simulink model "lss"  (R2022b)
settings: Solver=FixedStepAuto  StartTime=0.0  StopTime=Inf  FixedStep=0.001  RelTol=1e-3  EnableMultiTasking=on
InitFcn:
  | clear mex
model workspace (MAT data in the model file):
  worldsim_instance.endpoint_ip = '127.0.0.1'
  worldsim_instance.endpoint_port = 8080
values from neighbouring files (symbols this model uses):
  ADAS_Control_Mode = 1    [LSS_parameters.m]    (also in lss_ini_param.sldd = 1.0)
  butter_a = 1.0 -1.9911142922016536 0.99115359586893548    [lss_ini_param.sldd]
  butter_a_lka_out = 1.0 -1.5610180758007179 0.641351538057563    [lss_ini_param.sldd]
  butter_b = 9.825916820482009E-6 1.9651833640964018E-5 9.825916820482009E-6    [lss_ini_param.sldd]
  butter_b_lka_out = 0.020083365564211246 0.040166731128422492 0.020083365564211246    [lss_ini_param.sldd]
  index_variant_approaching_speed = 3.0    [lss_ini_param.sldd]
  initCond = vi_worldsim_load_scenario(worldsim_process,scenario_path,'lss_online')    [launcher.m]
  LDW_Activity_Flag = 1    [LSS_parameters.m]    (also in lss_ini_param.sldd = 1.0)
  LDW_Freq_Hz = Sensor_Freq_worldsim    [LSS_parameters.m]    (also in lss_ini_param.sldd = 50.0)
  LDW_LaneGap_dydt_Warning = 50    [LSS_parameters.m]    (also in lss_ini_param.sldd = 50.0)
  LDW_LaneGap_Warning = [0.5 0.25]    [LSS_parameters.m]    (also in lss_ini_param.sldd = 0.5 0.25)
  LDW_Min_Speed = 60    [LSS_parameters.m]    (also in lss_ini_param.sldd = 60.0)
  LDW_Steer_Vibration_Amplitude = 5    [LSS_parameters.m]    (also in lss_ini_param.sldd = 5.0)
  LDW_Steer_Vibration_Freq = 25    [LSS_parameters.m]    (also in lss_ini_param.sldd = 25.0)
  LKA_Activity_Flag = 1    [LSS_parameters.m]    (also in lss_ini_param.sldd = 1.0)
  LKA_D = [0.2 0.3]    [LSS_parameters.m]    (also in lss_ini_param.sldd = 0.2 0.3)
  LKA_Dyn_Rate_Limiter_Gain = 0.1    [LSS_parameters.m]    (also in lss_ini_param.sldd)
  LKA_Dyn_Rate_Limiter_Power = 10    [LSS_parameters.m]    (also in lss_ini_param.sldd = 10.0)
  LKA_Error_dydt_Off = 1    [LSS_parameters.m]    (also in lss_ini_param.sldd = 1.0)
  LKA_Error_Max = 3    [LSS_parameters.m]    (also in lss_ini_param.sldd = 3.0)
  LKA_Error_Off = 0.5    [LSS_parameters.m]    (also in lss_ini_param.sldd)
  LKA_Freq_Hz = Sensor_Freq_worldsim    [LSS_parameters.m]    (also in lss_ini_param.sldd = 50.0)
  LKA_I = [0.025 0.05]    [LSS_parameters.m]    (also in lss_ini_param.sldd = 0.025 0.05)
  LKA_Lane_Gap_Activate = [0.25 0.125]    [LSS_parameters.m]    (also in lss_ini_param.sldd = -0.05 0.125)
  LKA_Lane_Gap_dydt_Activate = 50    [LSS_parameters.m]    (also in lss_ini_param.sldd = 50.0)
  LKA_Min_Speed = 60    [LSS_parameters.m]    (also in lss_ini_param.mat = 50; lss_ini_param.sldd = 50.0)
  LKA_On_Display_Freq = 5    [LSS_parameters.m]    (also in lss_ini_param.sldd = 5.0)
  LKA_P = [0.1 0.2]    [LSS_parameters.m]    (also in lss_ini_param.sldd = 0.1 0.2)
  LKA_Steer_Rate_Max_radps = 1    [LSS_parameters.m]    (also in lss_ini_param.sldd = 1.0)
  radar_source = 2    [LSS_parameters.m]    (also in lss_ini_param.sldd = 2.0)
  Sensor_Freq_worldsim = 50    [launcher.m]    (also in lss_ini_param.sldd = 50.0)
  simulation_crt = '../VI-CarRealTime_model/SedanCar_WorldSim_Offline_send_svm.xml'    [launcher.m]
  stop_number_collisions = 5    [launcher.m]
  stop_speed = 0.001    [launcher.m]
  stop_time = 20    [launcher.m]
  target_speed = 72    [LSS_parameters.m]    (also in launcher.m = initCond.initialVelocity * 3.6)
  variant_approaching_speed = v_lat    [launcher.m]    (also in lss_ini_param.sldd = 0.2 0.3 0.4 0.5 0.6)
  vehicle_width = 1.86    [LSS_parameters.m]    (also in lss_ini_param.sldd = 2.05)
undefined symbols (not defined in the file or in its folder): Driver_Demands, light_brake_center, light_brake_left, light_brake_right, steer_assist, vicrt_initcallback, vicrt_initmexcallback, vicrt_simulationmanager
libraries: simulink x39, simwbSfunlib x15, viworldsim_lib x5
(part 1 of 6)
settings Model: Creator=mcava  LastModifiedBy=pumpaipa
settings SolverCC: AlgebraicLoopSolver=TrustRegion  AutoInsertRateTranBlk=on
settings DataIOCC: LimitDataPoints=on  SaveFormat=Array  ReturnWorkspaceOutputs=off  SignalLoggingName=sigsOut
settings OptimizationCC: ExpressionDepthLimit=2147483647  InitFltsAndDblsToZero=on  LifeSpan=inf
settings DebuggingCC: SignalInfNanChecking=warning  UnderspecifiedInitializationDetection=Classic  MergeDetectMultiDrivingBlocksExec=none  SignalResolutionControl=TryResolveAllWithWarning  MultiTaskDSMMsg=warning  MultiTaskCondExecSysMsg=none  FcnCallInpInsideContextMsg=warning  UnconnectedInputMsg=warning  UnconnectedOutputMsg=warning  UnconnectedLineMsg=warning  StateNameClashWarn=warning  SFUnexpectedBacktrackingDiag=warning  SFNoUnconditionalDefaultTransitionDiag=warning  SFExecutionAtInitializationDiag=none  SFMachineParentedDataDiag=warning  ArithmeticOperatorsInVariantConditions=warning
settings HardwareCC: ProdBitPerPointer=32  ProdBitPerSizeT=32  ProdBitPerPtrDiffT=32  ProdLargestAtomicFloat=None  ProdIntDivRoundTo=Undefined  ProdEndianess=Unspecified  ProdWordSize=32  ProdHWDeviceType=32-bit Generic  TargetHWDeviceType=32-bit Generic  TargetUnknown=on  ProdEqTarget=off
settings ModelReferenceCC: EnableRefExpFcnMdlSchedulingChecks=on  PropagateSignalLabelsOutOfModel=off
settings SFSimCC: SimUseLocalCustomCode=off  CustomCodeUndefinedFunction=UseInterfaceOnly
settings RTWCC: RTWUseLocalCustomCode=off
settings CodeAppCC: StateflowObjectComments=on
settings GRTTargetCC: TargetFcnLib=ansi_tfl_tmw.mat  TargetLangStandard=C89/C90 (ANSI)  CombineOutputUpdateFcns=off  GRTInterface=on
settings ConfigComp: CovMetricSettings=dw  CovSaveCumulativeToWorkspaceVar=on  CovSaveSingleToWorkspaceVar=on  CovExternalEMLEnable=off

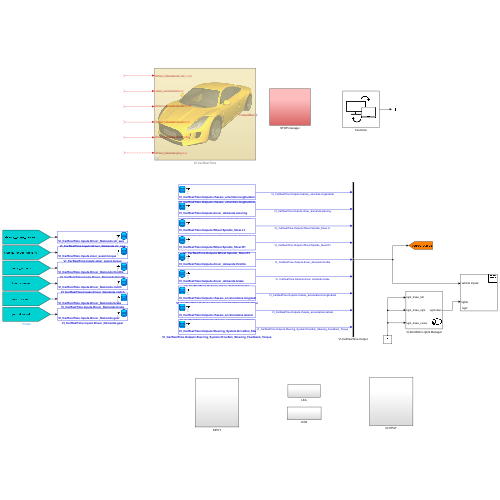
[thumbnail: Simulink's stored preview of the top-level diagram]
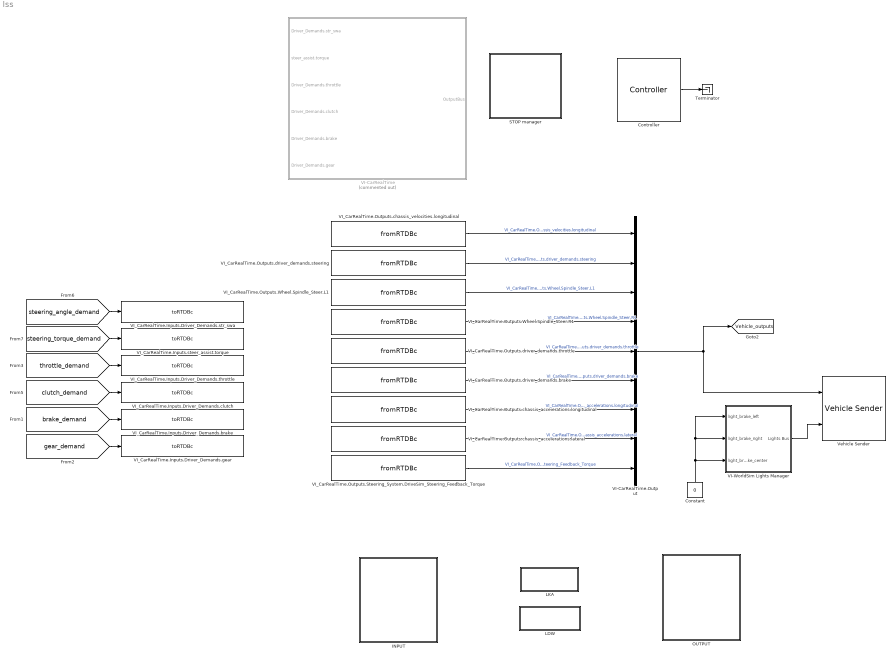
== system lss ==
  Constant : Constant  Value=0
  Controller : viworldsim_lib/Controller  worldsim_endpoint_ip=worldsim_instance.endpoint_ip  worldsim_endpoint_port=worldsim_instance.endpoint_port  worldsim_verbose=off
  INPUT : Subsystem
  LDW : Subsystem
  LKA : Subsystem
  OUTPUT : Subsystem
  STOP manager : Subsystem
  Terminator : Terminator
  VI-CarRealTime : Subsystem  Commented=on  InitFcn=vicrt_simulationmanager(0);  TreatAsAtomicUnit=on  mask{useOutputMapInMaskFlag=on}
      mask prompts: useOutputMapInMaskFlag "Output Port Names From Output Map"
      mask help: Full VI-CarRealTime mex integrated with IO Bus
      settings: CopyFcn=set_param(gcb, 'LinkStatus', 'none');  ModelCloseFcn=vicrt_simulationmanager(2);  OpenFcn=vicrt_simulationmanager(1);
      mask Display: image(imread('vehicle.jpg'));color('red');port_label('input',1,'Driver_Demands.str_swa');port_label('input',2,'steer_assist.torque');port_label('input',3,'Driver_Demands.throttle');port_label('input',4,'Driver_Demands.clutch');port_label('input',5,'Driver_Demands.brake');port_label('input',6,'Driver_Demands.gear');port_label('output',1,'OutputBus');
  VI-CarRealTime.Output : BusCreator  Inputs=9
  VI-WorldSim Lights Manager : Subsystem  mask{DummyMaskPar=0}
      mask init:
      | set_param(gcb, 'LinkStatus','none')
      settings: OpenFcn=|
      | wsoffline_lightsmanager;
      | set_param(gcb, 'LinkStatus','none');
      mask Display:
      | color('black');
      | image('lights.png', [85 0 50 50]);
  VI_CarRealTime.Inputs.Driver_Demands.brake : simwbSfunlib/toRTDBc  stringBlock=off  varName=VI_CarRealTime.Inputs.Driver_Demands.brake  sigDim=[1 1]  sigType=double  sampleTime=[-1 0]  maxBuffSize=1024  busName=nobus  defaultValue=0  defaultString=simwbout  hasMapping=0  ptrName=VI_CarRealTime_Inputs_Driver_Demands_brake  enumOrAlias=nothing
      settings: SourceProductName=SimWB MLToolkit
  VI_CarRealTime.Inputs.Driver_Demands.clutch : simwbSfunlib/toRTDBc  stringBlock=off  varName=VI_CarRealTime.Inputs.Driver_Demands.clutch  sigDim=[1 1]  sigType=double  sampleTime=[-1 0]  maxBuffSize=1024  busName=nobus  defaultValue=0  defaultString=simwbout  hasMapping=0  ptrName=VI_CarRealTime_Inputs_Driver_Demands_clutch  enumOrAlias=nothing
      settings: SourceProductName=SimWB MLToolkit
  VI_CarRealTime.Inputs.Driver_Demands.gear : simwbSfunlib/toRTDBc  stringBlock=off  varName=VI_CarRealTime.Inputs.Driver_Demands.gear  sigDim=[1 1]  sigType=double  sampleTime=[-1 0]  maxBuffSize=1024  busName=nobus  defaultValue=0  defaultString=simwbout  hasMapping=0  ptrName=VI_CarRealTime_Inputs_Driver_Demands_gear  enumOrAlias=nothing
      settings: SourceProductName=SimWB MLToolkit
  VI_CarRealTime.Inputs.Driver_Demands.str_swa : simwbSfunlib/toRTDBc  stringBlock=off  varName=VI_CarRealTime.Inputs.Driver_Demands.str_swa  sigDim=[1 1]  sigType=double  sampleTime=[-1 0]  maxBuffSize=1024  busName=nobus  defaultValue=0  defaultString=simwbout  hasMapping=0  ptrName=VI_CarRealTime_Inputs_Driver_Demands_str_swa  enumOrAlias=nothing
      settings: SourceProductName=SimWB MLToolkit
  VI_CarRealTime.Inputs.Driver_Demands.throttle : simwbSfunlib/toRTDBc  stringBlock=off  varName=VI_CarRealTime.Inputs.Driver_Demands.throttle  sigDim=[1 1]  sigType=double  sampleTime=[-1 0]  maxBuffSize=1024  busName=nobus  defaultValue=0  defaultString=simwbout  hasMapping=0  ptrName=VI_CarRealTime_Inputs_Driver_Demands_throttle  enumOrAlias=nothing
      settings: SourceProductName=SimWB MLToolkit
  VI_CarRealTime.Inputs.steer_assist.torque : simwbSfunlib/toRTDBc  stringBlock=off  varName=VI_CarRealTime.Inputs.steer_assist.torque  sigDim=[1 1]  sigType=double  sampleTime=[-1 0]  maxBuffSize=1024  busName=nobus  defaultValue=0  defaultString=simwbout  hasMapping=0  ptrName=VI_CarRealTime_Inputs_Driver_Demands_user_input_steering  enumOrAlias=nothing
      settings: SourceProductName=SimWB MLToolkit
  VI_CarRealTime.Outputs.Steering_System.DriveSim_Steering_Feedback_Torque : simwbSfunlib/fromRTDBc  stringBlock=off  varName=VI_CarRealTime.Outputs.Steering_System.DriveSim_Steering_Feedback_Torque  sigDim=[1 1]  sigType=double  sampleTime=[-1 0]  maxBuffSize=1024  busName=nobus  defaultValue=0  defaultString=simwbin  hasMapping=0  ptrName=VI_CarRealTime_Outputs_Steering_System_DriveSim_Steering_Feedback_Torque  enumOrAlias=nothing
      settings: SourceProductName=SimWB MLToolkit
  VI_CarRealTime.Outputs.Wheel.Spindle_Steer.L1 : simwbSfunlib/fromRTDBc  stringBlock=off  varName=VI_CarRealTime.Outputs.Wheel.Spindle_Steer.L1  sigDim=[1 1]  sigType=double  sampleTime=[-1 0]  maxBuffSize=1024  busName=nobus  defaultValue=0  defaultString=simwbin  hasMapping=0  ptrName=VI_CarRealTime_Outputs_Wheel_Spindle_Steer_L1  enumOrAlias=nothing
      settings: SourceProductName=SimWB MLToolkit
  VI_CarRealTime.Outputs.Wheel.Spindle_Steer.R1 : simwbSfunlib/fromRTDBc  stringBlock=off  varName=VI_CarRealTime.Outputs.Wheel.Spindle_Steer.R1  sigDim=[1 1]  sigType=double  sampleTime=[-1 0]  maxBuffSize=1024  busName=nobus  defaultValue=0  defaultString=simwbin  hasMapping=0  ptrName=VI_CarRealTime_Outputs_Wheel_Spindle_Steer_R1  enumOrAlias=nothing
      settings: SourceProductName=SimWB MLToolkit
  VI_CarRealTime.Outputs.chassis_accelerations.lateral : simwbSfunlib/fromRTDBc  stringBlock=off  varName=VI_CarRealTime.Outputs.chassis_accelerations.lateral  sigDim=[1 1]  sigType=double  sampleTime=[-1 0]  maxBuffSize=1024  busName=nobus  defaultValue=0  defaultString=simwbin  hasMapping=0  ptrName=VI_CarRealTime_Outputs_chassis_accelerations_lateral  enumOrAlias=nothing
      settings: SourceProductName=SimWB MLToolkit
  VI_CarRealTime.Outputs.chassis_accelerations.longitudinal : simwbSfunlib/fromRTDBc  stringBlock=off  varName=VI_CarRealTime.Outputs.chassis_accelerations.longitudinal  sigDim=[1 1]  sigType=double  sampleTime=[-1 0]  maxBuffSize=1024  busName=nobus  defaultValue=0  defaultString=simwbin  hasMapping=0  ptrName=VI_CarRealTime_Outputs_chassis_accelerations_longitudinal  enumOrAlias=nothing
      settings: SourceProductName=SimWB MLToolkit
  VI_CarRealTime.Outputs.chassis_velocities.longitudinal : simwbSfunlib/fromRTDBc  stringBlock=off  varName=VI_CarRealTime.Outputs.chassis_velocities.longitudinal  sigDim=[1 1]  sigType=double  sampleTime=[-1 0]  maxBuffSize=1024  busName=nobus  defaultValue=0  defaultString=simwbin  hasMapping=0  ptrName=VI_CarRealTime_Outputs_chassis_velocities_longitudinal  enumOrAlias=nothing
      settings: SourceProductName=SimWB MLToolkit
  VI_CarRealTime.Outputs.driver_demands.brake : simwbSfunlib/fromRTDBc  stringBlock=off  varName=VI_CarRealTime.Outputs.driver_demands.brake  sigDim=[1 1]  sigType=double  sampleTime=[-1 0]  maxBuffSize=1024  busName=nobus  defaultValue=0  defaultString=simwbin  hasMapping=0  ptrName=VI_CarRealTime_Outputs_driver_demands_brake  enumOrAlias=nothing
      settings: SourceProductName=SimWB MLToolkit
  VI_CarRealTime.Outputs.driver_demands.steering : simwbSfunlib/fromRTDBc  stringBlock=off  varName=VI_CarRealTime.Outputs.driver_demands.steering  sigDim=[1 1]  sigType=double  sampleTime=[-1 0]  maxBuffSize=1024  busName=nobus  defaultValue=0  defaultString=simwbin  hasMapping=0  ptrName=VI_CarRealTime_Outputs_driver_demands_steering  enumOrAlias=nothing
      settings: SourceProductName=SimWB MLToolkit
  VI_CarRealTime.Outputs.driver_demands.throttle : simwbSfunlib/fromRTDBc  stringBlock=off  varName=VI_CarRealTime.Outputs.driver_demands.throttle  sigDim=[1 1]  sigType=double  sampleTime=[-1 0]  maxBuffSize=1024  busName=nobus  defaultValue=0  defaultString=simwbin  hasMapping=0  ptrName=VI_CarRealTime_Outputs_driver_demands_throttle  enumOrAlias=nothing
      settings: SourceProductName=SimWB MLToolkit
  Vehicle Sender : viworldsim_lib/VI-WorldSim Vehicle Senders/Vehicle Sender  useOutputMapInMaskFlag=on  worldsim_car_name='ego'  worldsim_ai_controlled=off
  tag scope: Vehicle_outputs=global
  wires:
  VI-CarRealTime.Output/1 -> Vehicle Sender/1, [Vehicle_outputs]
  ? -> VI-CarRealTime/4(Driver_Demands.clutch)
  ? -> VI-CarRealTime/5(Driver_Demands.brake)
  ? -> VI-CarRealTime/2(steer_assist.torque)
  ? -> VI-CarRealTime/6(Driver_Demands.gear)
  ? -> VI-CarRealTime/3(Driver_Demands.throttle)
  ? -> VI-CarRealTime/1(Driver_Demands.str_swa)
  Controller/1 -> Terminator/1
  Constant/1 -> VI-WorldSim Lights Manager/3(light_brake_center), VI-WorldSim Lights Manager/2(light_brake_right), VI-WorldSim Lights Manager/1(light_brake_left)
  VI-WorldSim Lights Manager/1(Lights Bus) -> Vehicle Sender/2
  [steering_angle_demand] -> VI_CarRealTime.Inputs.Driver_Demands.str_swa/1
  [steering_torque_demand] -> VI_CarRealTime.Inputs.steer_assist.torque/1
  [throttle_demand] -> VI_CarRealTime.Inputs.Driver_Demands.throttle/1
  [clutch_demand] -> VI_CarRealTime.Inputs.Driver_Demands.clutch/1
  [brake_demand] -> VI_CarRealTime.Inputs.Driver_Demands.brake/1
  [gear_demand] -> VI_CarRealTime.Inputs.Driver_Demands.gear/1
  VI_CarRealTime.Outputs.Wheel.Spindle_Steer.R1/1 -> VI-CarRealTime.Output/4  "VI_CarRealTime.Outputs.Wheel.Spindle_Steer.R1"
  VI_CarRealTime.Outputs.chassis_velocities.longitudinal/1 -> VI-CarRealTime.Output/1  "VI_CarRealTime.Outputs.chassis_velocities.longitudinal"
  VI_CarRealTime.Outputs.Steering_System.DriveSim_Steering_Feedback_Torque/1 -> VI-CarRealTime.Output/9  "VI_CarRealTime.Outputs.Steering_System.DriveSim_Steering_Feedback_Torque"
  VI_CarRealTime.Outputs.chassis_accelerations.lateral/1 -> VI-CarRealTime.Output/8  "VI_CarRealTime.Outputs.chassis_accelerations.lateral"
  VI_CarRealTime.Outputs.driver_demands.brake/1 -> VI-CarRealTime.Output/6  "VI_CarRealTime.Outputs.driver_demands.brake"
  VI_CarRealTime.Outputs.Wheel.Spindle_Steer.L1/1 -> VI-CarRealTime.Output/3  "VI_CarRealTime.Outputs.Wheel.Spindle_Steer.L1"
  VI_CarRealTime.Outputs.driver_demands.throttle/1 -> VI-CarRealTime.Output/5  "VI_CarRealTime.Outputs.driver_demands.throttle"
  VI_CarRealTime.Outputs.driver_demands.steering/1 -> VI-CarRealTime.Output/2  "VI_CarRealTime.Outputs.driver_demands.steering"
  VI_CarRealTime.Outputs.chassis_accelerations.longitudinal/1 -> VI-CarRealTime.Output/7  "VI_CarRealTime.Outputs.chassis_accelerations.longitudinal"

== system lss/INPUT ==
  Inputs for CRT : Subsystem
  finalizing controls inputs : Subsystem
  simple_cruise_control : Subsystem

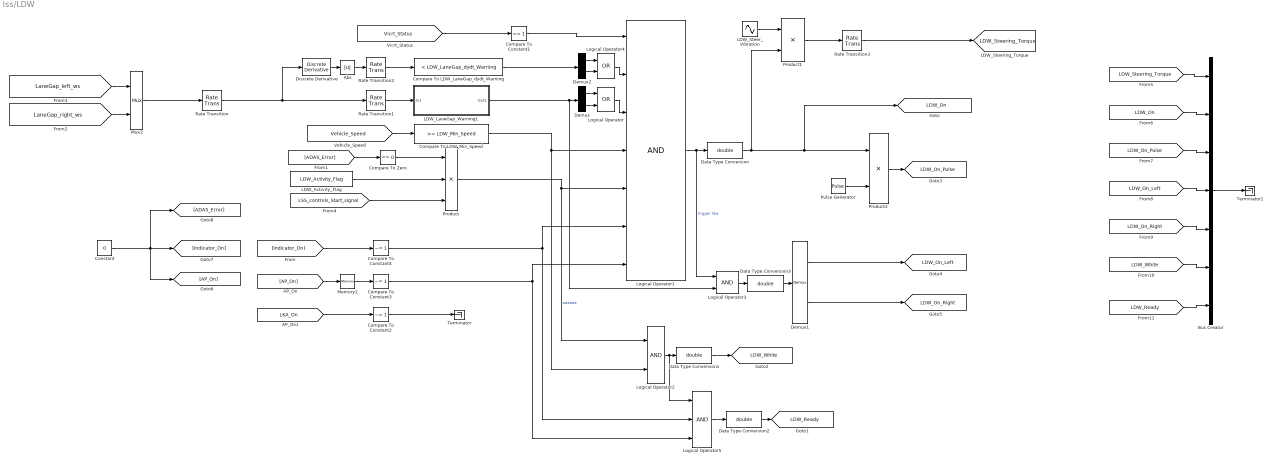
== system lss/LDW ==
  Abs : Abs  SaturateOnIntegerOverflow=off
  Bus Creator : BusCreator  Inputs=7
  Compare To Constant1 : simulink/Logic and Bit Operations/Compare To Constant  relop===  const=1  OutDataTypeStr=boolean
  Compare To Constant2 : simulink/Logic and Bit Operations/Compare To Constant  relop=~=  const=1  OutDataTypeStr=boolean
  Compare To Constant3 : simulink/Logic and Bit Operations/Compare To Constant  relop=~=  const=1  OutDataTypeStr=boolean
  Compare To Constant4 : simulink/Logic and Bit Operations/Compare To Constant  relop=~=  const=1  OutDataTypeStr=boolean
  Compare To Zero : simulink/Logic and Bit Operations/Compare To Zero  relop===  OutDataTypeStr=boolean
  Compare To LDW_LaneGap_dydt_Warning : simulink/Logic and Bit Operations/Compare To Constant  relop=<  const=LDW_LaneGap_dydt_Warning  OutDataTypeStr=boolean
  Compare To LDW_Min_Speed : simulink/Logic and Bit Operations/Compare To Constant  relop=>=  const=LDW_Min_Speed  OutDataTypeStr=boolean
  Constant : Constant  Value=0
  Data Type Conversion{,1..3} (4 alike) : DataTypeConversion  OutDataTypeStr=double  SaturateOnIntegerOverflow=off  RndMeth=Floor
  Demux : Demux  Outputs=2
  Demux1 : Demux  Outputs=2
  Demux2 : Demux  Outputs=2
  Discrete Derivative : simulink/Discrete/Discrete Derivative  gainval=1.0  ICPrevScaledInput=0.0  OutMin=[]  OutMax=[]  OutDataType=fixdt(1, 16)  OutScaling=2^-10  DoSatur=off
  LDW_Activity_Flag : Constant  Value=LDW_Activity_Flag
  LDW_LaneGap_Warning1 : Subsystem
  LDW_Steer_Vibration : Sin  Amplitude=LDW_Steer_Vibration_Amplitude  Frequency=LDW_Steer_Vibration_Freq*2*pi  SampleTime=0
  Logical Operator : Logic  Operator=OR  AllPortsSameDT=off  OutDataTypeStr=boolean
  Logical Operator1 : Logic  Inputs=7  AllPortsSameDT=off  OutDataTypeStr=boolean
  Logical Operator2 : Logic  AllPortsSameDT=off  OutDataTypeStr=boolean
  Logical Operator3 : Logic  AllPortsSameDT=off  OutDataTypeStr=boolean
  Logical Operator4 : Logic  Operator=OR  AllPortsSameDT=off  OutDataTypeStr=boolean
  Logical Operator5 : Logic  Inputs=3  AllPortsSameDT=off  OutDataTypeStr=boolean
  Memory2 : Memory
  Mux3 : Mux  Inputs=2
  Product : Product  Inputs=3
  Product1 : Product
  Product2 : Product
  Pulse Generator : DiscretePulseGenerator  PulseType=Time based  Period=1/LKA_On_Display_Freq  PulseWidth=50
  Rate Transition : RateTransition  OutPortSampleTime=1/LDW_Freq_Hz
  Rate Transition1 : RateTransition  OutPortSampleTime=1/1000
  Rate Transition2 : RateTransition  OutPortSampleTime=1/1000
  Rate Transition3 : RateTransition  OutPortSampleTime=1/1000
  Terminator : Terminator
  Terminator1 : Terminator
  tag scope: LDW_On=global, LDW_On_Left=global, LDW_On_Pulse=global, LDW_On_Right=global, LDW_Ready=global, LDW_Steering_Torque=global, LDW_White=global
  wires:
  [Vicrt_Status] -> Compare To Constant1/1
  Compare To Constant1/1 -> Logical Operator1/1
  Logical Operator1/1 -> Logical Operator3/1, Data Type Conversion/1  "trigger ldw"
  [Vehicle_Speed] -> Compare To LDW_Min_Speed/1
  Compare To LDW_Min_Speed/1 -> Logical Operator2/2, Logical Operator1/4
  Logical Operator/1 -> Logical Operator1/3
  LDW_Steer_Vibration/1 -> Product1/1
  Product1/1 -> Rate Transition3/1
  Data Type Conversion/1 -> Product2/1, [LDW_On], Product1/2
  Logical Operator2/1 -> Logical Operator5/1, Data Type Conversion1/1
  Data Type Conversion1/1 -> [LDW_White]
  Demux/1 -> Logical Operator/1
  Demux/2 -> Logical Operator/2
  Demux1/1 -> [LDW_On_Left]
  Demux1/2 -> [LDW_On_Right]
  Data Type Conversion3/1 -> Demux1/1
  Logical Operator3/1 -> Data Type Conversion3/1
  Rate Transition/1 -> Rate Transition1/1, Discrete Derivative/1
  Discrete Derivative/1 -> Abs/1
  Rate Transition2/1 -> Compare To LDW_LaneGap_dydt_Warning/1
  Compare To LDW_LaneGap_dydt_Warning/1 -> Demux2/1
  Logical Operator4/1 -> Logical Operator1/2
  Demux2/1 -> Logical Operator4/1
  Demux2/2 -> Logical Operator4/2
  Abs/1 -> Rate Transition2/1
  [Indicator_On] -> Compare To Constant4/1
  Compare To Constant4/1 -> Logical Operator1/6, Logical Operator5/2
  Logical Operator5/1 -> Data Type Conversion2/1
  Product/1 -> Logical Operator2/1, Logical Operator1/5  "aaaaaa"
  [ADAS_Error] -> Compare To Zero/1
  Compare To Zero/1 -> Product/1
  LDW_Activity_Flag/1 -> Product/2
  LDW_LaneGap_Warning1/1(Out1) -> Logical Operator3/2, Demux/1
  Rate Transition1/1 -> LDW_LaneGap_Warning1/1(In1)
  [AP_On] -> Memory2/1
  Memory2/1 -> Compare To Constant3/1
  Compare To Constant3/1 -> Logical Operator1/7, Logical Operator5/3
  Pulse Generator/1 -> Product2/2
  Product2/1 -> [LDW_On_Pulse]
  [LKA_On] -> Compare To Constant2/1
  Compare To Constant2/1 -> Terminator/1
  Rate Transition3/1 -> [LDW_Steering_Torque]
  Data Type Conversion2/1 -> [LDW_Ready]
  Mux3/1 -> Rate Transition/1
  [LaneGap_left_ws] -> Mux3/1
  [LaneGap_right_ws] -> Mux3/2
  [LSS_controls_Start_signal] -> Product/3
  Constant/1 -> [AP_On], [ADAS_Error], [Indicator_On]
  [LDW_Steering_Torque] -> Bus Creator/1
  [LDW_On] -> Bus Creator/2
  [LDW_On_Pulse] -> Bus Creator/3
  [LDW_On_Left] -> Bus Creator/4
  [LDW_On_Right] -> Bus Creator/5
  [LDW_White] -> Bus Creator/6
  [LDW_Ready] -> Bus Creator/7
  Bus Creator/1 -> Terminator1/1

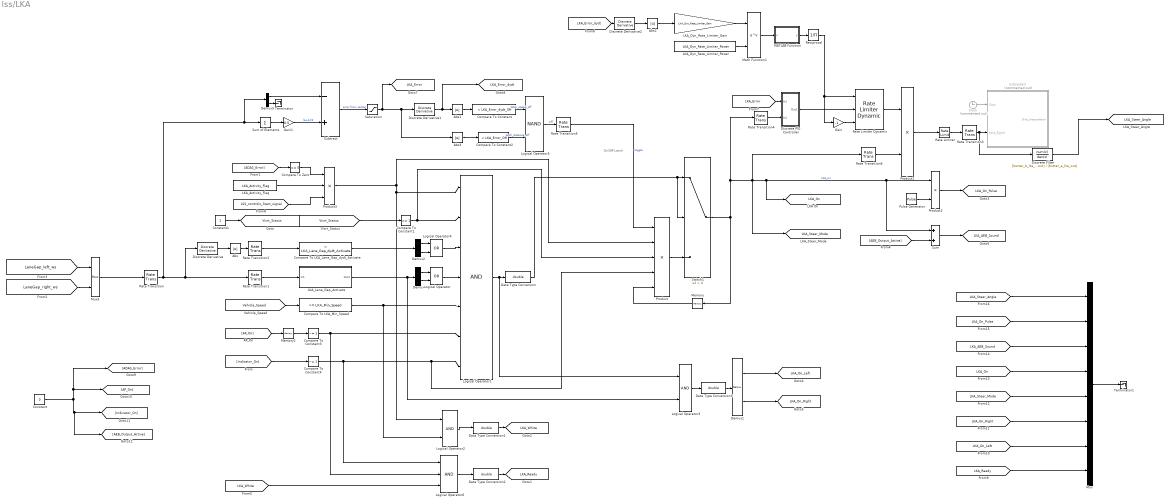
== system lss/LKA ==
  note: On/Off Latch
  Abs{,1..3} (4 alike) : Abs  SaturateOnIntegerOverflow=off
  Clock : Clock  Commented=on
  Compare To Constant : simulink/Logic and Bit Operations/Compare To Constant  relop=<  const=LKA_Error_dydt_Off  OutDataTypeStr=boolean
  Compare To Constant1 : simulink/Logic and Bit Operations/Compare To Constant  relop===  const=1  OutDataTypeStr=boolean
  Compare To Constant2 : simulink/Logic and Bit Operations/Compare To Constant  relop=<  const=LKA_Error_Off  OutDataTypeStr=boolean
  Compare To Constant3 : simulink/Logic and Bit Operations/Compare To Constant  relop=~=  const=1  OutDataTypeStr=boolean
  Compare To Constant4 : simulink/Logic and Bit Operations/Compare To Constant  relop=~=  const=1  OutDataTypeStr=boolean
  Compare To LKA_Lane_Gap_dydt_Activate : simulink/Logic and Bit Operations/Compare To Constant  relop=<  const=LKA_Lane_Gap_dydt_Activate  OutDataTypeStr=boolean
  Compare To LKA_Min_Speed : simulink/Logic and Bit Operations/Compare To Constant  relop=>=  const=LKA_Min_Speed  OutDataTypeStr=boolean
  Compare To Zero : simulink/Logic and Bit Operations/Compare To Zero  relop===  OutDataTypeStr=boolean
  Constant : Constant  Value=0
  Constant1 : Constant
  Data Type Conversion{,1..3} (4 alike) : DataTypeConversion  OutDataTypeStr=double  SaturateOnIntegerOverflow=off  RndMeth=Floor
  Demux{,1..3} (4 alike) : Demux  Outputs=2
  Discrete Derivative : simulink/Discrete/Discrete Derivative  gainval=1.0  ICPrevScaledInput=0.0  OutMin=[]  OutMax=[]  OutDataType=fixdt(1, 16)  OutScaling=2^-10  DoSatur=off
  Discrete Derivative1 : simulink/Discrete/Discrete Derivative  gainval=1.0  ICPrevScaledInput=0.0  OutMin=[]  OutMax=[]  OutDataType=fixdt(1, 16)  OutScaling=2^-10  DoSatur=off
  Discrete Derivative2 : simulink/Discrete/Discrete Derivative  gainval=1.0  ICPrevScaledInput=0.0  OutMin=[]  OutMax=[]  OutDataType=fixdt(1, 16)  OutScaling=2^-10  DoSatur=off
  Discrete Filter : DiscreteFilter  Numerator=[butter_b_lka_out]  Denominator=[butter_a_lka_out]  SampleTime=1e-3
  Discrete PID Controller : Subsystem
  Gain : Gain  Gain=-1
  Gain1 : Gain  Gain=0.5
  LKA_Activity_Flag : Constant  Value=LKA_Activity_Flag
  LKA_Dyn_Rate_Limiter_Gain : Gain  Gain=LKA_Dyn_Rate_Limiter_Gain
  LKA_Dyn_Rate_Limiter_Power : Constant  Value=LKA_Dyn_Rate_Limiter_Power
  LKA_Lane_Gap_Activate : Subsystem
  Logical Operator : Logic  Operator=OR  AllPortsSameDT=off  OutDataTypeStr=boolean
  Logical Operator1 : Logic  Inputs=7  AllPortsSameDT=off  OutDataTypeStr=boolean
  Logical Operator2 : Logic  AllPortsSameDT=off  OutDataTypeStr=boolean
  Logical Operator3 : Logic  AllPortsSameDT=off  OutDataTypeStr=boolean
  Logical Operator4 : Logic  Operator=OR  AllPortsSameDT=off  OutDataTypeStr=boolean
  Logical Operator5 : Logic  Operator=NAND  AllPortsSameDT=off  OutDataTypeStr=boolean
  Logical Operator6 : Logic  Inputs=3  AllPortsSameDT=off  OutDataTypeStr=boolean
  MATLAB Function : MATLAB Function  TreatAsAtomicUnit=on
  Math Function1 : Math  Operator=pow  SignedPower=on
  Memory : Memory
  Memory2 : Memory
  Mux : Mux  Inputs=8
  Mux3 : Mux  Inputs=2
  Product : Product  Inputs=5
  Product1 : Product
  Product2 : Product
  Product3 : Product  Inputs=3
  Pulse Generator : DiscretePulseGenerator  PulseType=Time based  Period=1/LKA_On_Display_Freq  PulseWidth=50
  Rate Limiter : RateLimiter  RisingSlewLimit=LKA_Steer_Rate_Max_radps  FallingSlewLimit=-LKA_Steer_Rate_Max_radps  SampleTimeMode=inherited
  Rate Limiter Dynamic : simulink/Discontinuities/Rate Limiter Dynamic
  Rate Transition : RateTransition  OutPortSampleTime=1/LKA_Freq_Hz
  Rate Transition{1..3,5} (4 alike) : RateTransition  OutPortSampleTime=1/1000
  Rate Transition4 : RateTransition  OutPortSampleTime=1/LKA_Freq_Hz
  Rate Transition6 : RateTransition  OutPortSampleTime=1/LKA_Freq_Hz
  Reciprocal : Product  Inputs=/  RndMeth=Zero  SaturateOnIntegerOverflow=on
  Saturation : Saturate  UpperLimit=LKA_Error_Max  LowerLimit=-LKA_Error_Max
  Subsystem : Subsystem  Commented=on
  Subtract : Sum  Inputs=-+
  Sum : Sum
  Sum of Elements : Sum  Inputs=+
  Switch1 : Switch  Criteria=u2 > Threshold  SaturateOnIntegerOverflow=off  InputSameDT=off
  Terminator : Terminator
  Terminator1 : Terminator
  tag scope: LKA_AEB_Sound=global, LKA_Error=global, LKA_Error_dydt=global, LKA_On=global, LKA_On_Left=global, LKA_On_Pulse=global, LKA_On_Right=global, LKA_Ready=global, LKA_Steer_Angle=global, LKA_Steer_Mode=global, LKA_White=global, Vicrt_Status=global
  wires:
  [Vicrt_Status] -> Compare To Constant1/1
  Compare To Constant1/1 -> Product/3, Logical Operator1/2
  Logical Operator1/1 -> Logical Operator3/1, Data Type Conversion/1
  [Vehicle_Speed] -> Compare To LKA_Min_Speed/1
  Compare To LKA_Min_Speed/1 -> Logical Operator1/5, Logical Operator2/2
  Logical Operator/1 -> Logical Operator1/4
  Logical Operator2/1 -> Data Type Conversion1/1
  Data Type Conversion1/1 -> [LKA_White]
  Demux/1 -> Logical Operator/1
  Demux/2 -> Logical Operator/2
  LKA_Lane_Gap_Activate/1(Out1) -> Logical Operator3/2, Demux/1
  Data Type Conversion3/1 -> Demux1/1
  Logical Operator3/1 -> Data Type Conversion3/1
  Rate Transition/1 -> Demux3/1, Sum of Elements/1, Discrete Derivative/1, Rate Transition1/1
  Discrete Derivative/1 -> Abs/1
  Rate Transition1/1 -> LKA_Lane_Gap_Activate/1(In1)
  Rate Transition2/1 -> Compare To LKA_Lane_Gap_dydt_Activate/1
  Compare To LKA_Lane_Gap_dydt_Activate/1 -> Demux2/1
  Logical Operator4/1 -> Logical Operator1/3
  Demux2/1 -> Logical Operator4/1
  Demux2/2 -> Logical Operator4/2
  Abs/1 -> Rate Transition2/1
  Data Type Conversion/1 -> Switch1/1, Switch1/2
  Product/1 -> Switch1/3
  Memory/1 -> Product/5
  Logical Operator5/1 -> Rate Transition5/1  "off"
  Sum of Elements/1 -> Gain1/1
  Gain1/1 -> Subtract/2  "(a+b)/2"
  Demux3/2 -> Terminator/1
  Demux3/1 -> Subtract/1
  Subtract/1 -> Saturation/1  "error from center"
  Clock/1 -> Subsystem/1(Clock)
  Compare To Constant/1 -> Logical Operator5/1  "latch_speed_off"
  Compare To Constant2/1 -> Logical Operator5/2  "latch_distance_off"
  Rate Transition5/1 -> Product/1  "toggle"
  Gain/1 -> Rate Limiter Dynamic/3
  Rate Limiter Dynamic/1 -> Product1/1
  Rate Limiter/1 -> Rate Transition3/1
  LKA_Dyn_Rate_Limiter_Power/1 -> Math Function1/2
  Math Function1/1 -> MATLAB Function/1(u)
  LKA_Dyn_Rate_Limiter_Gain/1 -> Math Function1/1
  Reciprocal/1 -> Rate Limiter Dynamic/1, Gain/1
  Abs1/1 -> Compare To Constant/1
  Discrete Derivative2/1 -> Abs2/1
  Abs2/1 -> LKA_Dyn_Rate_Limiter_Gain/1
  Abs3/1 -> Compare To Constant2/1
  Saturation/1 -> Abs3/1, Discrete Derivative1/1, [LKA_Error]
  Product1/1 -> Rate Limiter/1
  Rate Transition6/1 -> Product1/2
  Discrete Derivative1/1 -> Abs1/1, [LKA_Error_dydt]
  Pulse Generator/1 -> Product2/2
  Rate Transition3/1 -> Discrete Filter/1, Subsystem/2(Input_Signal)
  Mux3/1 -> Rate Transition/1
  [AP_On] -> Memory2/1
  Compare To Constant3/1 -> Logical Operator1/6, Logical Operator6/2
  Memory2/1 -> Compare To Constant3/1
  [Indicator_On] -> Compare To Constant4/1
  Compare To Constant4/1 -> Product/4, Logical Operator1/7, Logical Operator6/1
  Data Type Conversion2/1 -> [LKA_Ready]
  Logical Operator6/1 -> Data Type Conversion2/1
  [ADAS_Error] -> Compare To Zero/1
  Compare To Zero/1 -> Product3/1
  Product3/1 -> Logical Operator2/1, Logical Operator1/1, Product/2
  Rate Transition4/1 -> Discrete PID Controller/2(In2)
  Discrete PID Controller/1(Out1) -> Rate Limiter Dynamic/2
  Switch1/1 -> Rate Transition6/1, [LKA_Steer_Mode], [LKA_On], Sum/1, Product2/1, Rate Transition4/1, Memory/1  "LKA_on"
  [AEB_Output_Active] -> Sum/2
  Product2/1 -> [LKA_On_Pulse]
  Demux1/1 -> [LKA_On_Left]
  Demux1/2 -> [LKA_On_Right]
  Sum/1 -> [LKA_AEB_Sound]
  [LaneGap_right_ws] -> Mux3/2
  [LaneGap_left_ws] -> Mux3/1
  [LKA_White] -> Logical Operator6/3
  [LKA_Error_dydt] -> Discrete Derivative2/1
  [LKA_Error] -> Discrete PID Controller/1(In1)
  Constant1/1 -> [Vicrt_Status]
  Discrete Filter/1 -> [LKA_Steer_Angle]
  LKA_Activity_Flag/1 -> Product3/2
  [LSS_controls_Start_signal] -> Product3/3
  Constant/1 -> [AEB_Output_Active], [Indicator_On], [AP_On], [ADAS_Error]
  [LKA_Steer_Angle] -> Mux/1
  [LKA_On_Pulse] -> Mux/2
  [LKA_AEB_Sound] -> Mux/3
  [LKA_On] -> Mux/4
  [LKA_Steer_Mode] -> Mux/5
  [LKA_On_Right] -> Mux/6
  [LKA_On_Left] -> Mux/7
  [LKA_Ready] -> Mux/8
  Mux/1 -> Terminator1/1
  MATLAB Function/1(y) -> Reciprocal/1

== system lss/OUTPUT ==
  VI-CarRealTime_Outputs : Subsystem
  WorldSim_Sensor_Outputs : Subsystem
  rough data reporting : Subsystem

== system lss/STOP manager ==
  Clock2 : Clock
  Compare To Constant : simulink/Logic and Bit Operations/Compare To Constant  relop=>  const=stop_time  OutDataTypeStr=boolean
  Compare To Constant1 : simulink/Logic and Bit Operations/Compare To Constant  relop=<=  const=stop_speed  OutDataTypeStr=boolean
  Compare To Constant2 : simulink/Logic and Bit Operations/Compare To Constant  relop=>=  const=stop_number_collisions  OutDataTypeStr=boolean
  OR : Logic  Operator=OR  Inputs=4  AllPortsSameDT=off  OutDataTypeStr=boolean
  Stop Simulation : Stop
  wires:
  [collision_additive] -> Compare To Constant2/1
  Compare To Constant2/1 -> OR/3
  Compare To Constant/1 -> OR/1
  [Vehicle_Speed] -> Compare To Constant1/1
  Clock2/1 -> Compare To Constant/1
  Compare To Constant1/1 -> OR/2
  OR/1 -> Stop Simulation/1
  [LKA_Stop_signal] -> OR/4

== system lss/VI-CarRealTime ==
  Driver_Demands.str_swa : Inport
  steer_assist.torque : Inport  Port=2
  Driver_Demands.throttle : Inport  Port=3
  Driver_Demands.clutch : Inport  Port=4
  Driver_Demands.brake : Inport  Port=5
  Driver_Demands.gear : Inport  Port=6
  Input_Bus : Subsystem  LoadFcn=vicrt_initcallback(gcb);
      settings: CopyFcn=vicrt_initcallback(gcb);
  Output_Bus : Subsystem  Description=Outputs
      settings: CopyFcn=set_param(gcb, 'LinkStatus', 'none')
  vicrt_mex Standard : Subsystem  mask{vicrt_inputfile=simulation_crt, vicrt_outprefix='', intStep=0.001, AniFlag=off, inpPortDim=304, outPortDim=1377, NoDirectFeedthrough=on, AuxDataStruct=initCond, inpPortVecSize=0, outPortVecSize=0}
      mask prompts: vicrt_inputfile "VI-CarRealtime input file"; vicrt_outprefix "VI-CarRealTime output prefix"; intStep "Integration step"; AniFlag "live animation"; inpPortDim "input port dimension"; outPortDim "output port dimension"; NoDirectFeedthrough "Direct Feedthrough Off"; AuxDataStruct "Simulation Data Aux"; inpPortVecSize "Optional Vector Input Size"; outPortVecSize "Optional Vector Output Size"
      mask init:
      | custDriv=[1,1,1];
      settings: CopyFcn=set_param(gcb, 'LinkStatus', 'none')
  OutputBus : Outport  VectorParamsAs1DForOutWhenUnconnected=off
  wires:
  vicrt_mex Standard/1(Out1) -> Output_Bus/1(Outputs)
  Input_Bus/1(vicrt input) -> vicrt_mex Standard/1(In1)
  Driver_Demands.str_swa/1 -> Input_Bus/1(Driver_Demands.str_swa)
  steer_assist.torque/1 -> Input_Bus/2(steer_assist.torque)
  Driver_Demands.throttle/1 -> Input_Bus/3(Driver_Demands.throttle)
  Driver_Demands.clutch/1 -> Input_Bus/4(Driver_Demands.clutch)
  Driver_Demands.brake/1 -> Input_Bus/5(Driver_Demands.brake)
  Driver_Demands.gear/1 -> Input_Bus/6(Driver_Demands.gear)
  Output_Bus/1(OutputBus) -> OutputBus/1

== system lss/VI-WorldSim Lights Manager ==
  light_brake_left : Inport
  light_brake_right : Inport  Port=2
  light_brake_center : Inport  Port=3
  Lights : Subsystem
  Lights Bus : Outport  VectorParamsAs1DForOutWhenUnconnected=off
  wires:
  Lights/1(Out1) -> Lights Bus/1
  light_brake_left/1 -> Lights/1(light_brake_left)
  light_brake_right/1 -> Lights/2(light_brake_right)
  light_brake_center/1 -> Lights/3(light_brake_center)

== system lss/INPUT/Inputs for CRT ==
  Constant : Constant  Value=0
  Constant1 : Constant
  tag scope: brake_demand=global, clutch_demand=global, gear_demand=global, steering_angle_demand=global, steering_torque_demand=global, throttle_demand=global
  wires:
  Constant/1 -> [brake_demand]
  [LDW_Steering_Torque] -> [steering_torque_demand]
  [LKA_Steering_signal] -> [steering_angle_demand]
  [CC_throttle_demand] -> [clutch_demand]
  [CC_clutch_demand] -> [throttle_demand]
  Constant1/1 -> [gear_demand]

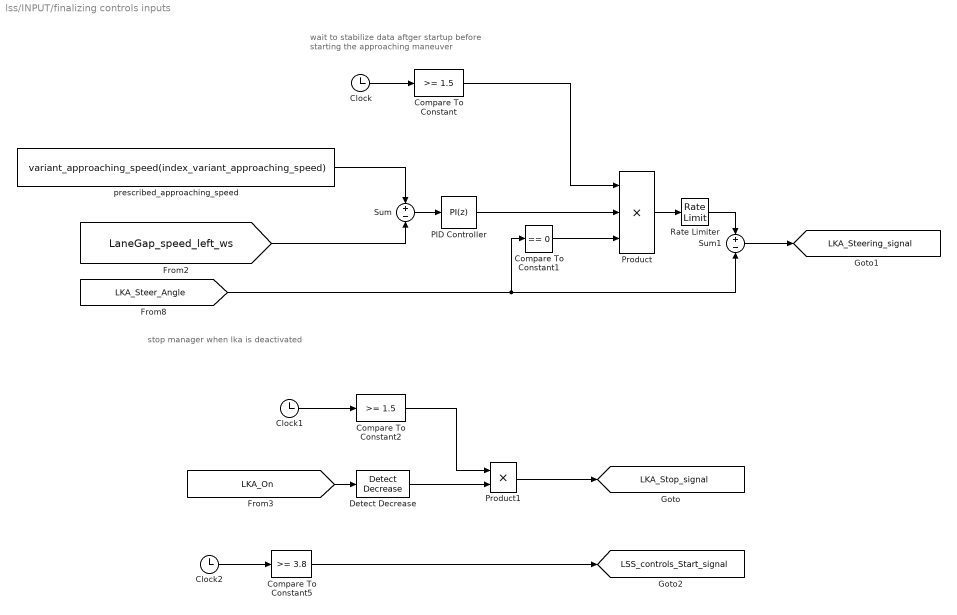
== system lss/INPUT/finalizing controls inputs ==
  note: stop manager when lka is deactivated
  note: wait to stabilize data aftger startup
      | before starting the approaching
      | maneuver
  Clock : Clock
  Clock1 : Clock
  Clock2 : Clock
  Compare To Constant : simulink/Logic and Bit Operations/Compare To Constant  relop=>=  const=1.5  OutDataTypeStr=boolean
  Compare To Constant1 : simulink/Logic and Bit Operations/Compare To Constant  relop===  const=0  OutDataTypeStr=boolean
  Compare To Constant2 : simulink/Logic and Bit Operations/Compare To Constant  relop=>=  const=1.5  OutDataTypeStr=boolean
  Compare To Constant5 : simulink/Logic and Bit Operations/Compare To Constant  relop=>=  const=3.8  OutDataTypeStr=boolean
  Detect Decrease : simulink/Logic and Bit Operations/Detect Decrease  vinit=0.0  OutDataTypeStr=boolean
  PID Controller : simulink/Continuous/PID Controller  Controller=PI  Form=Parallel  TimeDomain=Discrete-time  SampleTime=-1  IntegratorMethod=Forward Euler  FilterMethod=Forward Euler  ControllerParametersSource=internal  P=0.4  I=-0.002  D=0  UseFilter=on  N=100  TunerSelectOption=Transfer Function Based (PID Tuner App)  InitialConditionSource=internal  InitialConditionForIntegrator=0  InitialConditionForFilter=0  DifferentiatorICPrevScaledInput=0  ExternalReset=none  TrackingMode=off  Kt=1  LimitOutput=off  UpperSaturationLimit=inf  LowerSaturationLimit=-inf  LinearizeAsGain=on  AntiWindupMode=none  Kb=1  POutMin=[]  POutMax=[]  IOutMin=[]  IOutMax=[]  DOutMin=[]  DOutMax=[]  NOutMin=[]  NOutMax=[]  SumOutMin=[]  SumOutMax=[]  SaturationOutMin=[]  SaturationOutMax=[]  PParamMin=[]  PParamMax=[]  IParamMin=[]  IParamMax=[]  DParamMin=[]  DParamMax=[]  NParamMin=[]  NParamMax=[]  KbParamMin=[]  KbParamMax=[]  KtParamMin=[]  KtParamMax=[]  KbOutMin=[]  KbOutMax=[]  KtOutMin=[]  KtOutMax=[]  IntegratorOutMin=[]  IntegratorOutMax=[]  FilterOutMin=[]  FilterOutMax=[]  SumI1OutMin=[]  SumI1OutMax=[]  SumI2OutMin=[]  SumI2OutMax=[]  SumI3OutMin=[]  SumI3OutMax=[]  SumI4OutMin=[]  SumI4OutMax=[]  SumDOutMin=[]  SumDOutMax=[]  DifferentiatorOutMin=[]  DifferentiatorOutMax=[]  FilterDiffOutCoefMin=[]  FilterDiffOutCoefMax=[]  ReciprocalOutMin=[]  ReciprocalOutMax=[]  SumDenOutMin=[]  SumDenOutMax=[]  SumNumOutMin=[]  SumNumOutMax=[]  DivideOutMin=[]  DivideOutMax=[]  IntegratorContinuousStateAttributes=''  IntegratorStateMustResolveToSignalObject=off  IntegratorRTWStateStorageClass=Auto  FilterContinuousStateAttributes=''  FilterStateMustResolveToSignalObject=off  FilterRTWStateStorageClass=Auto  ParallelPVariant=InternalParameters  IdealPVariant=Disabled  IVariant=InternalParameters  DVariant=Disabled  IntegratorVariant=Discrete  SatVariant=Disabled  AWVariant=Passthrough  PCopyVariant=Disabled  TRVariant=Disabled  FdbkBlocksVariant=Forward  IdealPFdbkVariant=Disabled  SatFdbkVariant=Disabled  DerivativeFilterVariant=Disabled  NVariant=Disabled  NCopyVariant=Disabled_SignalSpec  FilterICVariant=Disabled  IntegratorICVariant=InternalICs  ExternalResetVariant=Disabled  TRSumVariant=Passthrough  SumFdbkVariant=Disabled  SumVariant=Sum_PI
  Product : Product  Inputs=3
  Product1 : Product
  Rate Limiter : RateLimiter  RisingSlewLimit=0.75  FallingSlewLimit=-inf  SampleTimeMode=inherited
  Sum : Sum  Inputs=+-
  Sum1 : Sum  Inputs=+-
  prescribed_approaching_speed : Constant  Value=variant_approaching_speed(index_variant_approaching_speed)
  tag scope: LKA_Steering_signal=global, LKA_Stop_signal=global, LSS_controls_Start_signal=global
  wires:
  Compare To Constant2/1 -> Product1/1
  [LaneGap_speed_left_ws] -> Sum/2
  Clock/1 -> Compare To Constant/1
  [LKA_Steer_Angle] -> Compare To Constant1/1, Sum1/2
  Product/1 -> Rate Limiter/1
  prescribed_approaching_speed/1 -> Sum/1
  Sum/1 -> PID Controller/1
  Compare To Constant1/1 -> Product/3
  Detect Decrease/1 -> Product1/2
  Compare To Constant/1 -> Product/1
  Sum1/1 -> [LKA_Steering_signal]
  Product1/1 -> [LKA_Stop_signal]
  PID Controller/1 -> Product/2
  Clock1/1 -> Compare To Constant2/1
  [LKA_On] -> Detect Decrease/1
  Compare To Constant5/1 -> [LSS_controls_Start_signal]
  Clock2/1 -> Compare To Constant5/1
  Rate Limiter/1 -> Sum1/1

== system lss/INPUT/simple_cruise_control ==
  note: This is used to mantaint the target speed until controller action
  Cast To Double : DataTypeConversion  OutDataTypeStr=double  SaturateOnIntegerOverflow=off  RndMeth=Floor
  Compare To Constant4 : simulink/Logic and Bit Operations/Compare To Constant  relop===  const=0  OutDataTypeStr=boolean
  Compare To Constant5 : simulink/Logic and Bit Operations/Compare To Constant  relop===  const=0  OutDataTypeStr=boolean
  Constant : Constant  Value=0
  PID Controller : simulink/Continuous/PID Controller  Controller=PI  Form=Parallel  TimeDomain=Discrete-time  SampleTime=-1  IntegratorMethod=Forward Euler  FilterMethod=Forward Euler  ControllerParametersSource=internal  P=40  I=10  D=0  UseFilter=on  N=100  TunerSelectOption=Transfer Function Based (PID Tuner App)  InitialConditionSource=internal  InitialConditionForIntegrator=0  InitialConditionForFilter=0  DifferentiatorICPrevScaledInput=0  ExternalReset=none  TrackingMode=off  Kt=1  LimitOutput=on  UpperSaturationLimit=100  LowerSaturationLimit=0  LinearizeAsGain=on  AntiWindupMode=none  Kb=1  POutMin=[]  POutMax=[]  IOutMin=[]  IOutMax=[]  DOutMin=[]  DOutMax=[]  NOutMin=[]  NOutMax=[]  SumOutMin=[]  SumOutMax=[]  SaturationOutMin=[]  SaturationOutMax=[]  PParamMin=[]  PParamMax=[]  IParamMin=[]  IParamMax=[]  DParamMin=[]  DParamMax=[]  NParamMin=[]  NParamMax=[]  KbParamMin=[]  KbParamMax=[]  KtParamMin=[]  KtParamMax=[]  KbOutMin=[]  KbOutMax=[]  KtOutMin=[]  KtOutMax=[]  IntegratorOutMin=[]  IntegratorOutMax=[]  FilterOutMin=[]  FilterOutMax=[]  SumI1OutMin=[]  SumI1OutMax=[]  SumI2OutMin=[]  SumI2OutMax=[]  SumI3OutMin=[]  SumI3OutMax=[]  SumI4OutMin=[]  SumI4OutMax=[]  SumDOutMin=[]  SumDOutMax=[]  DifferentiatorOutMin=[]  DifferentiatorOutMax=[]  FilterDiffOutCoefMin=[]  FilterDiffOutCoefMax=[]  ReciprocalOutMin=[]  ReciprocalOutMax=[]  SumDenOutMin=[]  SumDenOutMax=[]  SumNumOutMin=[]  SumNumOutMax=[]  DivideOutMin=[]  DivideOutMax=[]  IntegratorContinuousStateAttributes=''  IntegratorStateMustResolveToSignalObject=off  IntegratorRTWStateStorageClass=Auto  FilterContinuousStateAttributes=''  FilterStateMustResolveToSignalObject=off  FilterRTWStateStorageClass=Auto  ParallelPVariant=InternalParameters  IdealPVariant=Disabled  IVariant=InternalParameters  DVariant=Disabled  IntegratorVariant=Discrete  SatVariant=Enabled  AWVariant=Passthrough  PCopyVariant=Disabled  TRVariant=Disabled  FdbkBlocksVariant=Forward  IdealPFdbkVariant=Disabled  SatFdbkVariant=Disabled  DerivativeFilterVariant=Disabled  NVariant=Disabled  NCopyVariant=Disabled_SignalSpec  FilterICVariant=Disabled  IntegratorICVariant=InternalICs  ExternalResetVariant=Disabled  TRSumVariant=Passthrough  SumFdbkVariant=Disabled  SumVariant=Sum_PI
  Product : Product
  Sum : Sum  Inputs=+-
  target_speed_ : Constant  Value=target_speed
  tag scope: CC_clutch_demand=global, CC_throttle_demand=global
  wires:
  target_speed_/1 -> Sum/1
  Sum/1 -> PID Controller/1
  [Vehicle_Speed] -> Sum/2
  PID Controller/1 -> Product/1  "throttle"
  Product/1 -> Compare To Constant4/1, [CC_throttle_demand]
  Compare To Constant5/1 -> Product/2
  [AEB_Output_Brake] -> Compare To Constant5/1
  Compare To Constant4/1 -> Cast To Double/1
  Cast To Double/1 -> [CC_clutch_demand]
  Constant/1 -> [AEB_Output_Brake]

== system lss/LDW/LDW_LaneGap_Warning1 ==
  In1 : Inport
  ADAS_Control_Mode : Constant  Value=ADAS_Control_Mode
  LDW_LaneGap_Warning : Constant  Value=LDW_LaneGap_Warning(1)
  LDW_LaneGap_Warning1 : Constant  Value=LDW_LaneGap_Warning(2)  VectorParams1D=off
  Multiport Switch : MultiPortSwitch  Inputs=2  DataPortForDefault=Additional data port  DiagnosticForDefault=None  SaturateOnIntegerOverflow=off  InputSameDT=off
  Relational Operator : RelationalOperator  Operator=<  OutDataTypeStr=boolean  InputSameDT=off
  Out1 : Outport  VectorParamsAs1DForOutWhenUnconnected=off
  wires:
  ADAS_Control_Mode/1 -> Multiport Switch/1
  Multiport Switch/1 -> Relational Operator/2
  Relational Operator/1 -> Out1/1
  In1/1 -> Relational Operator/1
  LDW_LaneGap_Warning/1 -> Multiport Switch/4, Multiport Switch/2
  LDW_LaneGap_Warning1/1 -> Multiport Switch/3

== system lss/LKA/Discrete PID Controller ==
  In1 : Inport
  In2 : Inport  Port=2
  ADAS_Control_Mode : Constant  Value=ADAS_Control_Mode
  Demux : Demux  Outputs=3
  Discrete PID Controller : simulink/Continuous/PID Controller  Controller=PID  Form=Parallel  TimeDomain=Discrete-time  SampleTime=1/LKA_Freq_Hz  IntegratorMethod=Forward Euler  FilterMethod=Forward Euler  ControllerParametersSource=external  P=LKA_P  I=LKA_I  D=LKA_D  UseFilter=off  N=100  TunerSelectOption=Transfer Function Based (PID Tuner App)  InitialConditionSource=internal  InitialConditionForIntegrator=0  InitialConditionForFilter=0  DifferentiatorICPrevScaledInput=0  ExternalReset=either  TrackingMode=off  Kt=1  LimitOutput=off  UpperSaturationLimit=inf  LowerSaturationLimit=-inf  LinearizeAsGain=off  AntiWindupMode=clamping  Kb=1  POutMin=[]  POutMax=[]  IOutMin=[]  IOutMax=[]  DOutMin=[]  DOutMax=[]  NOutMin=[]  NOutMax=[]  SumOutMin=[]  SumOutMax=[]  SaturationOutMin=[]  SaturationOutMax=[]  PParamMin=[]  PParamMax=[]  IParamMin=[]  IParamMax=[]  DParamMin=[]  DParamMax=[]  NParamMin=[]  NParamMax=[]  KbParamMin=[]  KbParamMax=[]  KtParamMin=[]  KtParamMax=[]  KbOutMin=[]  KbOutMax=[]  KtOutMin=[]  KtOutMax=[]  IntegratorOutMin=[]  IntegratorOutMax=[]  FilterOutMin=[]  FilterOutMax=[]  SumI1OutMin=[]  SumI1OutMax=[]  SumI2OutMin=[]  SumI2OutMax=[]  SumI3OutMin=[]  SumI3OutMax=[]  SumI4OutMin=[]  SumI4OutMax=[]  SumDOutMin=[]  SumDOutMax=[]  DifferentiatorOutMin=[]  DifferentiatorOutMax=[]  FilterDiffOutCoefMin=[]  FilterDiffOutCoefMax=[]  ReciprocalOutMin=[]  ReciprocalOutMax=[]  SumDenOutMin=[]  SumDenOutMax=[]  SumNumOutMin=[]  SumNumOutMax=[]  DivideOutMin=[]  DivideOutMax=[]  IntegratorContinuousStateAttributes=''  IntegratorStateMustResolveToSignalObject=off  IntegratorRTWStateStorageClass=Auto  FilterContinuousStateAttributes=''  FilterStateMustResolveToSignalObject=off  FilterRTWStateStorageClass=Auto  ParallelPVariant=ExternalParameters  IdealPVariant=Disabled  IVariant=ExternalParameters  DVariant=ExternalParameters  IntegratorVariant=Discrete  SatVariant=Disabled  AWVariant=Passthrough  PCopyVariant=Disabled  TRVariant=Disabled  FdbkBlocksVariant=Forward  IdealPFdbkVariant=Disabled  SatFdbkVariant=Disabled  DerivativeFilterVariant=Differentiator  NVariant=Passthrough  NCopyVariant=Disabled_SignalSpec  FilterICVariant=InternalICsDifferentiator  IntegratorICVariant=InternalICs  ExternalResetVariant=ExternalReset  TRSumVariant=Passthrough  SumFdbkVariant=Disabled  SumVariant=Sum_PID
  LKA_D(1) : Constant  Value=LKA_D(1)
  LKA_D(1)1 : Constant  Value=LKA_D(2)
  LKA_I(1) : Constant  Value=LKA_I(1)
  LKA_I(1)1 : Constant  Value=LKA_I(2)
  LKA_P(1) : Constant  Value=LKA_P(1)
  LKA_P(1)1 : Constant  Value=LKA_P(2)
  Multiport Switch : MultiPortSwitch  Inputs=2  DataPortForDefault=Additional data port  DiagnosticForDefault=None  SaturateOnIntegerOverflow=off  InputSameDT=off
  Mux : Mux  Inputs=3
  Mux1 : Mux  Inputs=3
  Out1 : Outport  VectorParamsAs1DForOutWhenUnconnected=off
  wires:
  In1/1 -> Discrete PID Controller/1
  In2/1 -> Discrete PID Controller/5
  Discrete PID Controller/1 -> Out1/1
  LKA_P(1)/1 -> Mux/1
  ADAS_Control_Mode/1 -> Multiport Switch/1
  Demux/2 -> Discrete PID Controller/3
  Demux/3 -> Discrete PID Controller/4
  Demux/1 -> Discrete PID Controller/2
  Mux1/1 -> Multiport Switch/3
  Mux/1 -> Multiport Switch/4, Multiport Switch/2
  LKA_I(1)/1 -> Mux/2
  LKA_D(1)/1 -> Mux/3
  LKA_P(1)1/1 -> Mux1/1
  LKA_I(1)1/1 -> Mux1/2
  LKA_D(1)1/1 -> Mux1/3
  Multiport Switch/1 -> Demux/1

== system lss/LKA/LKA_Lane_Gap_Activate ==
  In1 : Inport
  ADAS_Control_Mode : Constant  Value=ADAS_Control_Mode
  LKA_Lane_Gap_Activate : Constant  Value=LKA_Lane_Gap_Activate(1)
  LKA_Lane_Gap_Activate2 : Constant  Value=LKA_Lane_Gap_Activate(2)  VectorParams1D=off
  Multiport Switch : MultiPortSwitch  Inputs=2  DataPortForDefault=Additional data port  DiagnosticForDefault=None  SaturateOnIntegerOverflow=off  InputSameDT=off
  Relational Operator : RelationalOperator  Operator=<  OutDataTypeStr=boolean  InputSameDT=off
  Out1 : Outport  VectorParamsAs1DForOutWhenUnconnected=off
  wires:
  ADAS_Control_Mode/1 -> Multiport Switch/1
  Multiport Switch/1 -> Relational Operator/2
  Relational Operator/1 -> Out1/1
  In1/1 -> Relational Operator/1
  LKA_Lane_Gap_Activate/1 -> Multiport Switch/4, Multiport Switch/2
  LKA_Lane_Gap_Activate2/1 -> Multiport Switch/3

== system lss/LKA/Subsystem ==
  Clock : Inport
  Input_Signal : Inport  Port=2
  Delay : Delay  DelayLength=1000/LKA_Freq_Hz  InitialCondition=-1/LKA_Freq_Hz
  Delay1 : Delay  DelayLength=1000/LKA_Freq_Hz
  Delay2 : Delay  DelayLength=1000/LKA_Freq_Hz
  Lookup Table Dynamic : simulink/Lookup Tables/Lookup Table Dynamic  LookUpMeth=Interpolation-Use End Values  OutDataType=fixdt('double')  OutScaling=[]  OutputDataTypeScalingMode=Specify via dialog  OutDataTypeStr=fixdt('double')  DoSatur=off
  Vector Concatenate : Concatenate
  Vector Concatenate1 : Concatenate
  Zero-Order Hold1 : ZeroOrderHold  SampleTime=1/LKA_Freq_Hz
  Zero-Order Hold2 : ZeroOrderHold  SampleTime=1/LKA_Freq_Hz
  Zero-Order Hold3 : ZeroOrderHold  SampleTime=1e-3
  Zero-Order Hold4 : ZeroOrderHold  SampleTime=1e-3
  1kHz_Interpolation : Outport  VectorParamsAs1DForOutWhenUnconnected=off
  wires:
  Input_Signal/1 -> Zero-Order Hold1/1
  Zero-Order Hold1/1 -> Zero-Order Hold4/1
  Zero-Order Hold3/1 -> Delay/1, Vector Concatenate/2
  Zero-Order Hold2/1 -> Zero-Order Hold3/1
  Delay/1 -> Vector Concatenate/1
  Delay1/1 -> Lookup Table Dynamic/1
  Delay2/1 -> Vector Concatenate1/1
  Zero-Order Hold4/1 -> Delay2/1, Vector Concatenate1/2
  Vector Concatenate1/1 -> Lookup Table Dynamic/3
  Vector Concatenate/1 -> Lookup Table Dynamic/2
  Clock/1 -> Delay1/1, Zero-Order Hold2/1
  Lookup Table Dynamic/1 -> 1kHz_Interpolation/1

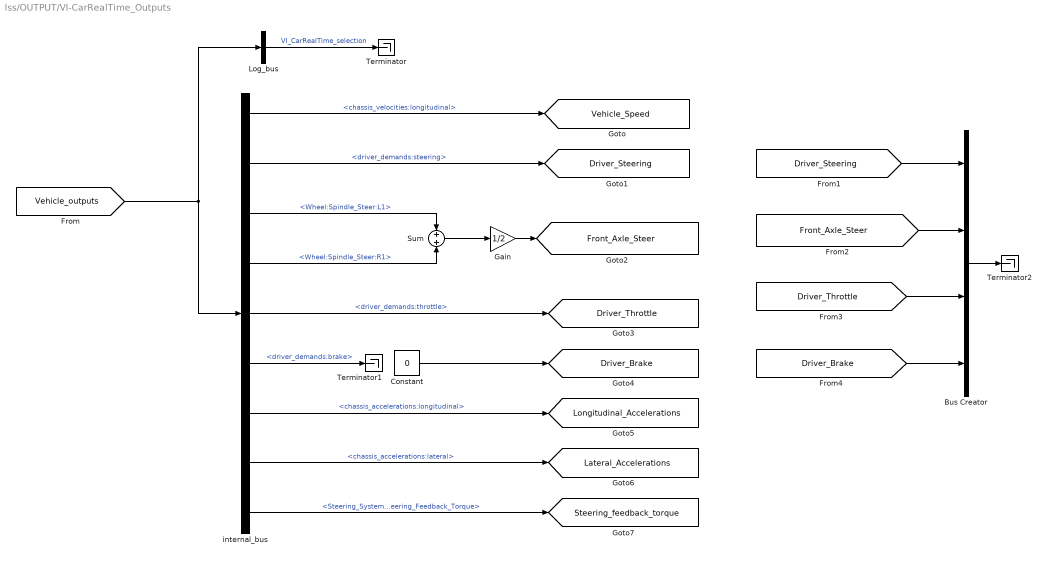
== system lss/OUTPUT/VI-CarRealTime_Outputs ==
  Bus Creator : BusCreator  Inputs=4
  Constant : Constant  Value=0
  Gain : Gain  Gain=1/2
  Log_bus : BusSelector  OutputSignals=chassis_velocities:longitudinal,chassis_accelerations:longitudinal,driver_demands:brake,driver_demands:throttle,driver_demands:steering,transmission:gear,engine:engine_rpm,chassis_accelerations:lateral,chassis_accelerations:vertical,chassis_velocities:lateral,chassis_velocities:pitch,chassis_velocities:roll,chassis_velocities:vertical,chassis_velocities:yaw,Steering_Column:steering_assist_force,Steering_System:DriveSim_Steering_Feedback_Torque  OutputAsBus=on
  Sum : Sum
  Terminator : Terminator
  Terminator1 : Terminator
  Terminator2 : Terminator
  internal_bus : BusSelector  OutputSignals=chassis_velocities:longitudinal,driver_demands:steering,Wheel:Spindle_Steer:L1,Wheel:Spindle_Steer:R1,driver_demands:throttle,driver_demands:brake,chassis_accelerations:longitudinal,chassis_accelerations:lateral,Steering_System:DriveSim_Steering_Feedback_Torque
  tag scope: Driver_Brake=global, Driver_Steering=global, Driver_Throttle=global, Front_Axle_Steer=global, Lateral_Accelerations=global, Longitudinal_Accelerations=global, Steering_feedback_torque=global, Vehicle_Speed=global
  wires:
  internal_bus/1 -> [Vehicle_Speed]  "<chassis_velocities:longitudinal>"
  Log_bus/1 -> Terminator/1  "VI_CarRealTime_selection"
  internal_bus/2 -> [Driver_Steering]  "<driver_demands:steering>"
  [Vehicle_outputs] -> Log_bus/1, internal_bus/1
  internal_bus/3 -> Sum/1  "<Wheel:Spindle_Steer:L1>"
  internal_bus/4 -> Sum/2  "<Wheel:Spindle_Steer:R1>"
  Sum/1 -> Gain/1
  Gain/1 -> [Front_Axle_Steer]
  internal_bus/5 -> [Driver_Throttle]  "<driver_demands:throttle>"
  Constant/1 -> [Driver_Brake]
  internal_bus/6 -> Terminator1/1  "<driver_demands:brake>"
  internal_bus/7 -> [Longitudinal_Accelerations]  "<chassis_accelerations:longitudinal>"
  internal_bus/8 -> [Lateral_Accelerations]  "<chassis_accelerations:lateral>"
  internal_bus/9 -> [Steering_feedback_torque]  "<Steering_System:DriveSim_Steering_Feedback_Torque>"
  [Driver_Steering] -> Bus Creator/1
  [Front_Axle_Steer] -> Bus Creator/2
  [Driver_Throttle] -> Bus Creator/3
  [Driver_Brake] -> Bus Creator/4
  Bus Creator/1 -> Terminator2/1
